simulink model "temperature"  (R2020b)
settings: Solver=VariableStepAuto  StartTime=0.0  StopTime=10.0  MaxStep=1  MinStep=1  RelTol=1e-3
model workspace: external: MATLAB File /Users/xinbo/MATLAB/projects/I o T/house_data.m (data not in the file)
undefined symbols (not defined in the file): c, M, Req
settings Model: Creator=xinbo  LastModifiedBy=xinbo

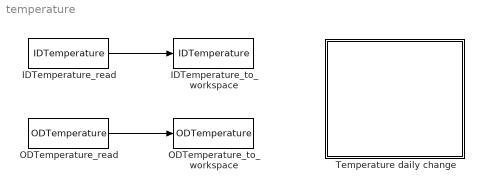
== system temperature ==
  IDTemperature_read : DataStoreRead  DataStoreName=IDTemperature
  IDTemperature_to_workspace : ToWorkspace  VariableName=IDTemperature  SampleTime=-1
      settings: Save2DSignal=2-D array (concatenate along first dimension)
  ODTemperature_read : DataStoreRead  DataStoreName=ODTemperature
  ODTemperature_to_workspace : ToWorkspace  VariableName=ODTemperature  SampleTime=-1
      settings: Save2DSignal=2-D array (concatenate along first dimension)
  Temperature daily change : Subsystem
      mask Display: image('/Users/xinbo/E/paper3/program_clean/digital_twin/images/temperature.png'); % Use "Edit Image" on toolstrip to change.
  wires:
  IDTemperature_read/1 -> IDTemperature_to_workspace/1
  ODTemperature_read/1 -> ODTemperature_to_workspace/1

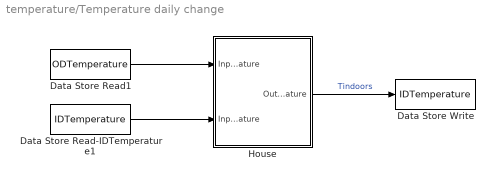
== system temperature/Temperature daily change ==
  Data Store Read-IDTemperature1 : DataStoreRead  DataStoreName=IDTemperature
  Data Store Read1 : DataStoreRead  DataStoreName=ODTemperature
  Data Store Write : DataStoreWrite  DataStoreName=IDTemperature
  House : Subsystem
      mask Display: image('/Users/xinbo/E/paper3/program_clean/digital_twin/images/home.png'); % Use "Edit Image" on toolstrip to change.
  wires:
  Data Store Read-IDTemperature1/1 -> House/2(Input-IDTemperature)
  Data Store Read1/1 -> House/1(Input-ODTemperature)
  House/1(Output-IDTemperature) -> Data Store Write/1  "Tindoors"

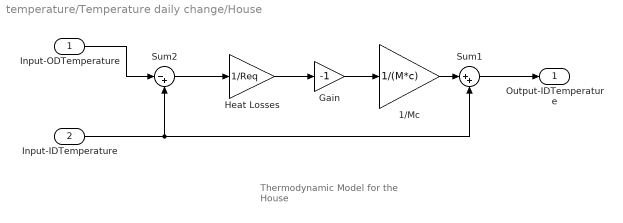
== system temperature/Temperature daily change/House ==
  note: Thermodynamic Model
      | for the House
  Input-ODTemperature : Inport
  Input-IDTemperature : Inport  Port=2
  1/Mc : Gain  Gain=1/(M*c)  SaturateOnIntegerOverflow=on  OutDataTypeStr=Inherit: Same as input  ParamDataTypeStr=Inherit: Same as input
  Gain : Gain  Gain=-1
  Heat Losses : Gain  Gain=1/Req  SaturateOnIntegerOverflow=on  OutDataTypeStr=Inherit: Same as input  ParamDataTypeStr=Inherit: Same as input
  Sum1 : Sum  Inputs=|++  InputSameDT=on  SaturateOnIntegerOverflow=on  OutDataTypeStr=Inherit: Same as first input
  Sum2 : Sum  Inputs=|-+  InputSameDT=on  SaturateOnIntegerOverflow=on  OutDataTypeStr=Inherit: Same as first input
  Output-IDTemperature : Outport  InitialOutput=0  VectorParamsAs1DForOutWhenUnconnected=off
  wires:
  Input-ODTemperature/1 -> Sum2/1
  Gain/1 -> 1/Mc/1
  Sum2/1 -> Heat Losses/1
  Heat Losses/1 -> Gain/1
  1/Mc/1 -> Sum1/1
  Sum1/1 -> Output-IDTemperature/1
  Input-IDTemperature/1 -> Sum1/2, Sum2/2
